simulink model "Q_3_3_Inertia_Estimation"  (R2024b)
settings: Solver=VariableStepAuto  StartTime=0.0  StopTime=20  RelTol=1e-3
InitFcn:
  | load_params_inertial_case
  | PID_calculations
values from neighbouring files (symbols this model uses):
  delta_c = 1 / sqrt(2)    [PID_calculations.m]
  delta_i = 1 / sqrt(2)    [PID_calculations.m]
  K_D = K_P * T_D    [PID_calculations.m]
  K_I = K_P / T_I    [PID_calculations.m]
  K_P = DeltaK * cos(DeltaPhi)    [PID_calculations.m]
  T_L = 5 * w_gc    [PID_calculations.m]
  w_c = 2 * pi * 20    (= 125.663706144)    [PID_calculations.m]
  w_ci = 2 * pi * 20    (= 125.663706144)    [PID_calculations.m]
undefined symbols (not defined in the file or in its folder): gbox, mot, rads2rpm, rpm2rads, sens
settings Model: Creator=JS  LastModifiedBy=JS
settings DebuggingCC: AlgebraicLoopMsg=none

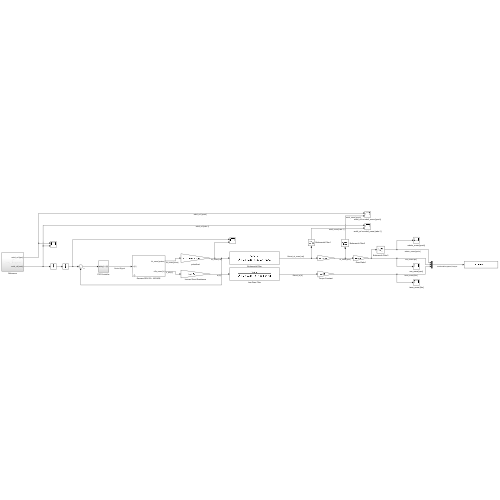
[thumbnail: Simulink's stored preview of the top-level diagram]
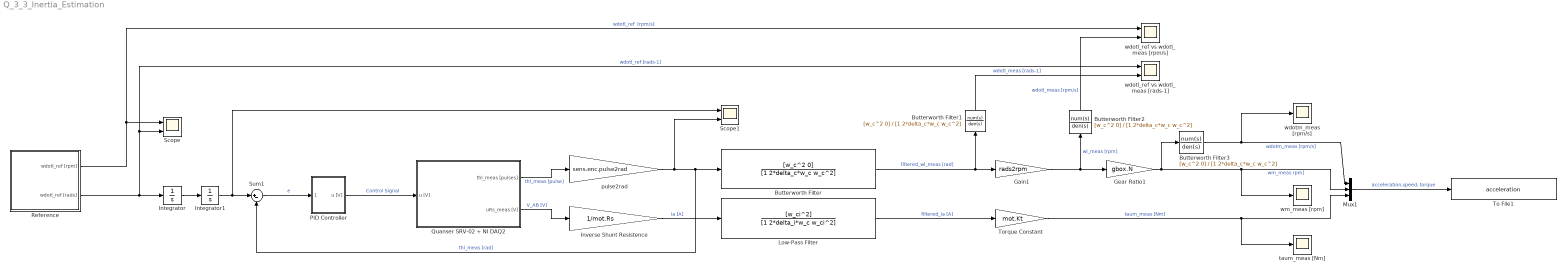
== system Q_3_3_Inertia_Estimation ==
  " taum_meas [Nm]" : Scope
  Butterworth Filter{,1..3} (4 alike) : TransferFcn  Numerator=[w_c^2 0]  Denominator=[1 2*delta_c*w_c w_c^2]
  Gain1 : Gain  Gain=rads2rpm
  Gear Ratio1 : Gain  Gain=gbox.N
  Integrator : Integrator
  Integrator1 : Integrator
  Inverse Shunt Resistence : Gain  Gain=1/mot.Rs
  Low-Pass Filter : TransferFcn  Numerator=[w_ci^2]  Denominator=[1 2*delta_i*w_c w_ci^2]
  Mux1 : Mux  Inputs=3
  PID Controller : Subsystem
  Quanser SRV-02 + NI DAQ2 : Subsystem  mask(Quanser SRV-02 (with inertial load) + NI DAQ){Ts=0.001, fricType=Coulomb + viscous}
      mask prompts: Ts "NI DAQ Sample Time:"; fricType "Friction model"
      mask help: Quanser SRV-02 (with inertial load) + NI DAQ model.
      mask init:
      | %%  Sensors data
      | 
      | %   shunt resistor
      | sens.curr.Rs = 0.5;                         %   resistance [Ohm]   
      | sens.curr.uRs_std = 0.01;                   %   voltage noise standard dev [V]                           
      | sens.curr.uRs_var = sens.curr.uRs_std^2;	%   voltage noise variance [V^2]
      | 
      | %   Hewlett-Packard HEDS-5540#A06 optical encoder
      | sens.enc.ppr = 500*4;                       %   pulses per rotation
      | sens.enc.pulse2deg = 360/sens.enc.ppr;      %   [pulses] -> [deg]
      | sens.enc.pulse2rad = 2*pi/sens.enc.ppr;     %   [pulses] -> [rad]
      | sens.enc.deg2pulse = sens.enc.ppr/360;      %   [deg] -> [pulses]
      | sens.enc.rad2pulse = sens.enc.ppr/2/pi;     %   [rad] -> [pulses]
      | 
      | 
      | %%  Data acquisition board (daq) data
      | 
      | %   NI PCI-6221 DAC data
      | daq.dac.bits = 16;                                  %   resolution (bits)
      | daq.dac.fs   = 10;                                  %   full scale 
      | daq.dac.q    = 2*daq.dac.fs/(2^daq.dac.bits-1);     %	quantization
      | 
      | %   NI PCI-6221 ADC data
      | daq.adc.bits = 16;                                  %   resolution (bits)
      | daq.adc.fs   = 10;                                  %   full scale (as set in SLDRT Analog Input block)
      | daq.adc.q    = 2*daq.adc.fs/(2^daq.adc.bits-1);     %   quantization
      mask Help:
      | Riccardo Antonello (antonello@dei.unipd.it)
      | 
      | April 24, 2020
      | 
      | Dept. of Information Engineering, University of Padova
      mask TypeOptions fricType: Coulomb + viscous | Karnopp
  Reference : Subsystem
  Scope : Scope  NumInputPorts=2
  Scope1 : Scope  NumInputPorts=2
  Sum1 : Sum  Inputs=|+-
  To File1 : ToFile  Filename=acceleration  MatrixName=acceleration  SaveFormat=Timeseries
  Torque Constant : Gain  Gain=mot.Kt
  pulse2rad : Gain  Gain=sens.enc.pulse2rad
  wdotl_ref vs wdotl_meas [rads-1] : Scope  NumInputPorts=2
  wdotl_ref vs wdotl_meas [rpm/s] : Scope  NumInputPorts=2
  wdotm_meas [rpm/s] : Scope
  wm_meas [rpm] : Scope
  wires:
  Reference/1(wdotl_ref [rpm]) -> Scope/1, wdotl_ref vs wdotl_meas [rpm/s]/1  "wdotl_ref  [rpm/s]"
  Quanser SRV-02 + NI DAQ2/1(thl_meas [pulses]) -> pulse2rad/1  "thl_meas [pulse]"
  Sum1/1 -> PID Controller/1(e[deg])  "e"
  Butterworth Filter/1 -> Butterworth Filter1/1, Gain1/1  "filtered_wl_meas [rad]"
  Reference/2(wdotl_ref [rads]) -> wdotl_ref vs wdotl_meas [rads-1]/1, Scope/2, Integrator/1  "wdotl_ref [rads-1]"
  Gear Ratio1/1 -> Mux1/2, wm_meas [rpm]/1, Butterworth Filter3/1  "wm_meas rpm]"
  Low-Pass Filter/1 -> Torque Constant/1  "filtered_ia [A]"
  Torque Constant/1 -> Mux1/3, " taum_meas [Nm]"/1  "taum_meas [Nm]"
  Quanser SRV-02 + NI DAQ2/2(uRs_meas [V]) -> Inverse Shunt Resistence/1  "V_AB [V]"
  Gain1/1 -> Gear Ratio1/1, Butterworth Filter2/1  "wl_meas [rpm]"
  pulse2rad/1 -> Scope1/2, Sum1/2, Butterworth Filter/1  "thl_meas [rad]"
  Mux1/1 -> To File1/1  "acceleration,speed, torque"
  Inverse Shunt Resistence/1 -> Low-Pass Filter/1  "ia [A]"
  PID Controller/1(u [V]) -> Quanser SRV-02 + NI DAQ2/1(u [V])  "Control Signal"
  Integrator1/1 -> Sum1/1, Scope1/1
  Integrator/1 -> Integrator1/1
  Butterworth Filter2/1 -> wdotl_ref vs wdotl_meas [rpm/s]/2  "wdotl_meas [rpm/s]"
  Butterworth Filter1/1 -> wdotl_ref vs wdotl_meas [rads-1]/2  "wdotl_meas [rads-1]"
  Butterworth Filter3/1 -> Mux1/1, wdotm_meas [rpm/s]/1  "wdotm_meas [rpm/s]"

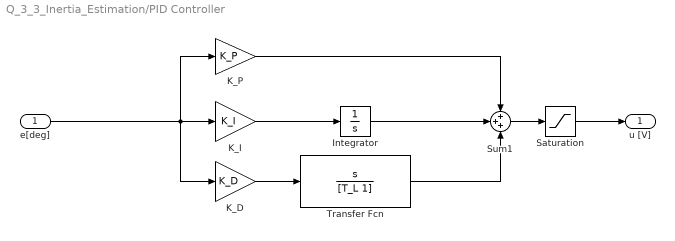
== system Q_3_3_Inertia_Estimation/PID Controller ==
  e[deg] : Inport
  Integrator : Integrator  ZeroCross=off
  K_D : Gain  Gain=K_D
  K_I : Gain  Gain=K_I
  K_P : Gain  Gain=K_P
  Saturation : Saturate  UpperLimit=10  LowerLimit=-10
  Sum1 : Sum  Inputs=+++
  Transfer Fcn : TransferFcn  Numerator=[1 0]  Denominator=[T_L 1]
  u [V] : Outport
  wires:
  Sum1/1 -> Saturation/1
  e[deg]/1 -> K_P/1, K_D/1, K_I/1
  K_D/1 -> Transfer Fcn/1
  Integrator/1 -> Sum1/2
  Saturation/1 -> u [V]/1
  K_I/1 -> Integrator/1
  Transfer Fcn/1 -> Sum1/3
  K_P/1 -> Sum1/1

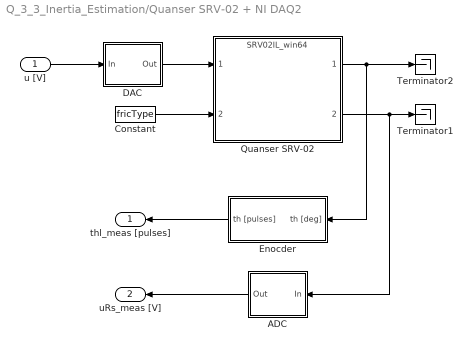
== system Q_3_3_Inertia_Estimation/Quanser SRV-02 + NI DAQ2 ==
  u [V] : Inport
  ADC : Subsystem
  Constant : Constant  Value=fricType
  DAC : Subsystem
  Enocder : Subsystem
  Quanser SRV-02 : ModelReference  ModelNameDialog=SRV02IL_win64.slxp  ModelReferenceVersion=1.44  CopyOfModelProtected=on
  Terminator1 : Terminator
  Terminator2 : Terminator
  thl_meas [pulses] : Outport
  uRs_meas [V] : Outport  Port=2
  wires:
  Enocder/1(th [pulses]) -> thl_meas [pulses]/1
  ADC/1(Out) -> uRs_meas [V]/1
  DAC/1(Out) -> Quanser SRV-02/1
  Quanser SRV-02/2 -> ADC/1(In), Terminator1/1
  u [V]/1 -> DAC/1(In)
  Quanser SRV-02/1 -> Enocder/1(th [deg]), Terminator2/1
  Constant/1 -> Quanser SRV-02/2

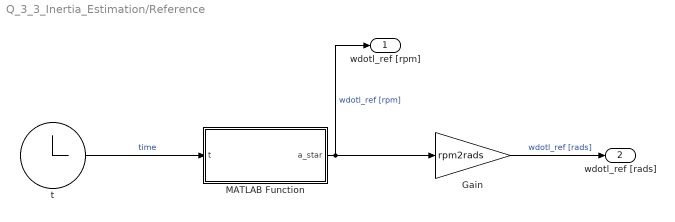
== system Q_3_3_Inertia_Estimation/Reference ==
  Gain : Gain  Gain=rpm2rads
  MATLAB Function : MATLAB Function  TreatAsAtomicUnit=on
  t : Clock
  wdotl_ref [rpm] : Outport
  wdotl_ref [rads] : Outport  Port=2
  wires:
  MATLAB Function/1(a_star) -> wdotl_ref [rpm]/1, Gain/1  "wdotl_ref [rpm]"
  t/1 -> MATLAB Function/1(t)  "time"
  Gain/1 -> wdotl_ref [rads]/1  "wdotl_ref [rads]"

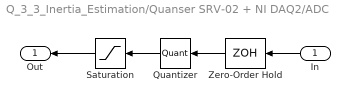
== system Q_3_3_Inertia_Estimation/Quanser SRV-02 + NI DAQ2/ADC ==
  In : Inport
  Quantizer : Quantizer  QuantizationInterval=daq.adc.q
  Saturation : Saturate  UpperLimit=daq.adc.fs  LowerLimit=-daq.adc.fs
  Zero-Order Hold : ZeroOrderHold  SampleTime=Ts
  Out : Outport
  wires:
  Saturation/1 -> Out/1
  In/1 -> Zero-Order Hold/1
  Quantizer/1 -> Saturation/1
  Zero-Order Hold/1 -> Quantizer/1

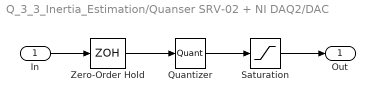
== system Q_3_3_Inertia_Estimation/Quanser SRV-02 + NI DAQ2/DAC ==
  In : Inport
  Quantizer : Quantizer  QuantizationInterval=daq.dac.q
  Saturation : Saturate  UpperLimit=daq.dac.fs  LowerLimit=-daq.dac.fs
  Zero-Order Hold : ZeroOrderHold  SampleTime=Ts
  Out : Outport
  wires:
  Quantizer/1 -> Saturation/1
  In/1 -> Zero-Order Hold/1
  Zero-Order Hold/1 -> Quantizer/1
  Saturation/1 -> Out/1

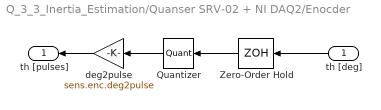
== system Q_3_3_Inertia_Estimation/Quanser SRV-02 + NI DAQ2/Enocder ==
  th [deg] : Inport
  Quantizer : Quantizer  QuantizationInterval=sens.enc.pulse2deg
  Zero-Order Hold : ZeroOrderHold  SampleTime=Ts
  deg2pulse : Gain  Gain=sens.enc.deg2pulse
  th [pulses] : Outport
  wires:
  Quantizer/1 -> deg2pulse/1
  th [deg]/1 -> Zero-Order Hold/1
  Zero-Order Hold/1 -> Quantizer/1
  deg2pulse/1 -> th [pulses]/1

== matlab function Q_3_3_Inertia_Estimation/Reference/MATLAB Function ==
  data: t input; a_star output
function a_star = acceleration_reference(t)
    % Simulink-compatible function block
    A = 450; % Amplitude (rpm/s)
    delta_T = 1; % Duration of each acceleration/deceleration phase (s)
    
    % Compute acceleration profile
    k = floor(t / delta_T);
    a_star = ((-1).^k) * A;
end
